simulink model "VB_RIFKF_UWB_INS25"  (R2023a)
settings: Solver=FixedStepAuto  StartTime=0.0  StopTime=500  FixedStep=0.01  RelTol=1e-3
InitFcn:
  | resilient_initNavigation1216;
  | init_param;
  | param_bias;
undefined symbols (not defined in the file or in its folder): dt, g0, gam0_rad, ISUS_flag, lp_GPS_sample_time, lp_Lidar_knoise, lp_Lidar_max, lp_Lidar_min, lp_Lidar_sample_time, lp_Lidar_seed, lp_UWB_knoise, lp_UWB_sample_time, lp_UWB_seed, lp_UWB_XY_max, lp_UWB_XY_min, magnitude, p, P0, P0_RIEKF, param, pd0, pe0, phi0_rad, pn0, psi, psi0_rad, state_dim, vd0, ve0, vn0
libraries: simulink_extras x108, simulink x89, dspstat3 x74, sharedtransform x61, matrix_library x11, sharedTrackingLibrary x8, aerolibconvert2 x5, aerolibtransform2 x5, dspfactors x3
(part 17 of 29)

== system VB_RIFKF_UWB_INS25/相对传感器模拟3/Subsystem/laser model ==
  note: 方位角测量白噪声均方根 ：0.1°
  psi & theta : Inport
  Bus Creator : BusCreator  Inputs=2
  Demux : Demux  Outputs=2
  Zero-Order Hold1 : ZeroOrderHold  SampleTime=lp_GPS_sample_time
  Zero-Order Hold2 : ZeroOrderHold  SampleTime=lp_GPS_sample_time
  bias & noise z1 : Subsystem  mask(Bias and Noise Model){noise_min=lp_Lidar_min, noise_max=lp_Lidar_max, noise_seed=lp_Lidar_seed, noise_k=lp_Lidar_knoise, sample_time=lp_Lidar_sample_time}
      mask prompts: noise_min "Minimum of the noise:"; noise_max "Maximum of the noise:"; noise_seed "Seed of the noise:"; noise_k "Noise coefficiet:"; sample_time "Sample time"
  bias & noise z3 : Subsystem  mask(Bias and Noise Model){noise_min=lp_Lidar_min, noise_max=lp_Lidar_max, noise_seed=lp_Lidar_seed, noise_k=lp_Lidar_knoise, sample_time=lp_Lidar_sample_time}
      mask prompts: noise_min "Minimum of the noise:"; noise_max "Maximum of the noise:"; noise_seed "Seed of the noise:"; noise_k "Noise coefficiet:"; sample_time "Sample time"
  psi out : Outport
  wires:
  Zero-Order Hold2/1 -> bias & noise z1/1(normal)  "theta13"
  Zero-Order Hold1/1 -> bias & noise z3/1(normal)  "theta12"
  Bus Creator/1 -> psi out/1
  bias & noise z3/1(real) -> Bus Creator/1  "psi12_k"
  bias & noise z1/1(real) -> Bus Creator/2  "psi12_k-1"
  psi & theta/1 -> Demux/1
  Demux/1 -> Zero-Order Hold1/1
  Demux/2 -> Zero-Order Hold2/1

== system VB_RIFKF_UWB_INS25/相对传感器模拟3/Subsystem2/radar model ==
  note: 相对距离测量白噪声均方根：3m
  r_xyz : Inport
  Bus Creator : BusCreator  Inputs=2
  Demux : Demux  Outputs=2
  Subsystem1 : Subsystem
  Zero-Order Hold1 : ZeroOrderHold  SampleTime=lp_GPS_sample_time
  Zero-Order Hold2 : ZeroOrderHold  SampleTime=lp_GPS_sample_time
  bias & noise x : Subsystem  mask(Bias and Noise Model){noise_min=lp_UWB_XY_min, noise_max=lp_UWB_XY_max, noise_seed=lp_UWB_seed, noise_k=lp_UWB_knoise, sample_time=lp_UWB_sample_time}
      mask prompts: noise_min "Minimum of the noise:"; noise_max "Maximum of the noise:"; noise_seed "Seed of the noise:"; noise_k "Noise coefficiet:"; sample_time "Sample time"
  bias & noise x1 : Subsystem  mask(Bias and Noise Model){noise_min=lp_UWB_XY_min, noise_max=lp_UWB_XY_max, noise_seed=lp_UWB_seed, noise_k=lp_UWB_knoise, sample_time=lp_UWB_sample_time}
      mask prompts: noise_min "Minimum of the noise:"; noise_max "Maximum of the noise:"; noise_seed "Seed of the noise:"; noise_k "Noise coefficiet:"; sample_time "Sample time"
  r_xyz out : Outport
  wires:
  Zero-Order Hold2/1 -> bias & noise x1/1(normal)  "r13"
  Zero-Order Hold1/1 -> bias & noise x/1(normal)  "r12"
  bias & noise x1/1(real) -> Subsystem1/1(u)
  bias & noise x/1(real) -> Bus Creator/1  "r12_k"
  Demux/2 -> Zero-Order Hold2/1
  Demux/1 -> Zero-Order Hold1/1
  r_xyz/1 -> Demux/1
  Bus Creator/1 -> r_xyz out/1
  Subsystem1/1(y) -> Bus Creator/2  "r12_k-1"

== system VB_RIFKF_UWB_INS25/相对传感器模拟4/Subsystem/laser model ==
  note: 方位角测量白噪声均方根 ：0.1°
  psi & theta : Inport
  Bus Creator : BusCreator  Inputs=2
  Demux : Demux  Outputs=2
  Zero-Order Hold1 : ZeroOrderHold  SampleTime=lp_GPS_sample_time
  Zero-Order Hold2 : ZeroOrderHold  SampleTime=lp_GPS_sample_time
  bias & noise z1 : Subsystem  mask(Bias and Noise Model){noise_min=lp_Lidar_min, noise_max=lp_Lidar_max, noise_seed=lp_Lidar_seed, noise_k=lp_Lidar_knoise, sample_time=lp_Lidar_sample_time}
      mask prompts: noise_min "Minimum of the noise:"; noise_max "Maximum of the noise:"; noise_seed "Seed of the noise:"; noise_k "Noise coefficiet:"; sample_time "Sample time"
  bias & noise z3 : Subsystem  mask(Bias and Noise Model){noise_min=lp_Lidar_min, noise_max=lp_Lidar_max, noise_seed=lp_Lidar_seed, noise_k=lp_Lidar_knoise, sample_time=lp_Lidar_sample_time}
      mask prompts: noise_min "Minimum of the noise:"; noise_max "Maximum of the noise:"; noise_seed "Seed of the noise:"; noise_k "Noise coefficiet:"; sample_time "Sample time"
  psi out : Outport
  wires:
  Demux/2 -> Zero-Order Hold2/1
  Demux/1 -> Zero-Order Hold1/1
  psi & theta/1 -> Demux/1
  bias & noise z1/1(real) -> Bus Creator/2  "psi12_k-1"
  bias & noise z3/1(real) -> Bus Creator/1  "psi12_k"
  Bus Creator/1 -> psi out/1
  Zero-Order Hold1/1 -> bias & noise z3/1(normal)  "theta12"
  Zero-Order Hold2/1 -> bias & noise z1/1(normal)  "theta13"

== system VB_RIFKF_UWB_INS25/相对传感器模拟4/Subsystem2/radar model ==
  note: 相对距离测量白噪声均方根：3m
  r_xyz : Inport
  Bus Creator : BusCreator  Inputs=2
  Demux : Demux  Outputs=2
  Subsystem1 : Subsystem
  Zero-Order Hold1 : ZeroOrderHold  SampleTime=lp_GPS_sample_time
  Zero-Order Hold2 : ZeroOrderHold  SampleTime=lp_GPS_sample_time
  bias & noise x : Subsystem  mask(Bias and Noise Model){noise_min=lp_UWB_XY_min, noise_max=lp_UWB_XY_max, noise_seed=lp_UWB_seed, noise_k=lp_UWB_knoise, sample_time=lp_UWB_sample_time}
      mask prompts: noise_min "Minimum of the noise:"; noise_max "Maximum of the noise:"; noise_seed "Seed of the noise:"; noise_k "Noise coefficiet:"; sample_time "Sample time"
  bias & noise x1 : Subsystem  mask(Bias and Noise Model){noise_min=lp_UWB_XY_min, noise_max=lp_UWB_XY_max, noise_seed=lp_UWB_seed, noise_k=lp_UWB_knoise, sample_time=lp_UWB_sample_time}
      mask prompts: noise_min "Minimum of the noise:"; noise_max "Maximum of the noise:"; noise_seed "Seed of the noise:"; noise_k "Noise coefficiet:"; sample_time "Sample time"
  r_xyz out : Outport
  wires:
  Subsystem1/1(y) -> Bus Creator/2  "r12_k-1"
  Bus Creator/1 -> r_xyz out/1
  r_xyz/1 -> Demux/1
  Demux/1 -> Zero-Order Hold1/1
  Demux/2 -> Zero-Order Hold2/1
  bias & noise x/1(real) -> Bus Creator/1  "r12_k"
  bias & noise x1/1(real) -> Subsystem1/1(u)
  Zero-Order Hold1/1 -> bias & noise x/1(normal)  "r12"
  Zero-Order Hold2/1 -> bias & noise x1/1(normal)  "r13"

== system VB_RIFKF_UWB_INS25/ER EKF M1/Error State Kalman Filter/Extended Kalman Filter1/Correct1 ==
  yMeas : Inport  SampleTime=SampleTime
  R : Inport  Port=2  SampleTime=SampleTime
  uMeas : Inport  Port=3  SampleTime=SampleTime
  uBlockOrdering : Inport  Port=4  SampleTime=SampleTime
  Enable : EnablePort
  Correct : MATLAB Function  TreatAsAtomicUnit=on
  Data Store ReadP : DataStoreRead  DataStoreName=P  IndexOptions=Index vector (dialog)  Indices=1  OutputSizes=1
  Data Store ReadX : DataStoreRead  DataStoreName=x  IndexOptions=Index vector (dialog)  Indices=1  OutputSizes=1
  Data Store WriteP : DataStoreWrite  DataStoreName=P  IndexOptions=Index vector (dialog)  Indices=1  OutputSizes=1
  Data Store WriteX : DataStoreWrite  DataStoreName=x  IndexOptions=Index vector (dialog)  Indices=1  OutputSizes=1
  RegisterSimulinkFcn : S-Function  FunctionName=ekfukfRegisterSimulinkFcn  Parameters=int32(3), 1, pM.HasAdditiveNoise, SampleTime, DataType, SLFcnsToRegister  SFunctionDeploymentMode=off  EnableBusSupport=off
  Scope : Scope
  Sk_m_innovation : Subsystem
  yBlockOrdering : Outport  VectorParamsAs1DForOutWhenUnconnected=off
  wires:
  Data Store ReadX/1 -> Sk_m_innovation/3(X), RegisterSimulinkFcn/1, Correct/1(x)
  Data Store ReadP/1 -> Sk_m_innovation/1(Pk/k_1), Correct/2("P ")
  Correct/2(P) -> Data Store WriteP/1
  R/1 -> Sk_m_innovation/4(R), Correct/4(R), RegisterSimulinkFcn/3
  Correct/1(xNew) -> Data Store WriteX/1
  Correct/3(blockOrdering) -> yBlockOrdering/1
  uBlockOrdering/1 -> Correct/6("blockOrdering ")
  uMeas/1 -> Correct/5(uMeas)
  yMeas/1 -> Sk_m_innovation/2(yMeas), RegisterSimulinkFcn/2, Correct/3(yMeas)
  Sk_m_innovation/1(measurement innovation) -> Scope/1

== system VB_RIFKF_UWB_INS25/ER EKF M1/Error State Kalman Filter/Extended Kalman Filter1/Output ==
  uBlockOrdering : Inport
  Data Store Read : DataStoreRead  DataStoreName=x  IndexOptions=Index vector (dialog)  Indices=1  OutputSizes=1
  Data Store Read1 : DataStoreRead  DataStoreName=P  IndexOptions=Index vector (dialog)  Indices=1  OutputSizes=1
  MATLAB Function : MATLAB Function  TreatAsAtomicUnit=on
  x : Outport  VectorParamsAs1DForOutWhenUnconnected=off
  P : Outport  Port=2  VectorParamsAs1DForOutWhenUnconnected=off
  yBlockOrdering : Outport  Port=3  VectorParamsAs1DForOutWhenUnconnected=off
  wires:
  Data Store Read/1 -> x/1
  Data Store Read1/1 -> MATLAB Function/1(S)
  uBlockOrdering/1 -> yBlockOrdering/1
  MATLAB Function/1(P) -> P/1

== system VB_RIFKF_UWB_INS25/ER EKF M1/Error State Kalman Filter/Extended Kalman Filter1/Predict ==
  Q : Inport  SampleTime=SampleTime
  uState : Inport  Port=2  SampleTime=SampleTime
  uBlockOrdering : Inport  Port=3  SampleTime=SampleTime
  Data Store Read1 : DataStoreRead  Commented=on  DataStoreName=feedback_flag_18dim  IndexOptions=Index vector (dialog)  Indices=1  OutputSizes=1
  Data Store Write : DataStoreWrite  DataStoreName=P  IndexOptions=Index vector (dialog)  Indices=1  OutputSizes=1
  Data Store Write1 : DataStoreWrite  DataStoreName=x  IndexOptions=Index vector (dialog)  Indices=1  OutputSizes=1
  Data Store WriteX : DataStoreWrite  DataStoreName=x  IndexOptions=Index vector (dialog)  Indices=1  OutputSizes=1
  Data Store ReadP : DataStoreRead  DataStoreName=P  IndexOptions=Index vector (dialog)  Indices=1  OutputSizes=1
  Data Store ReadX : DataStoreRead  DataStoreName=x  IndexOptions=Index vector (dialog)  Indices=1  OutputSizes=1
  If : If  Commented=on  IfExpression=u1 == 1  ShowElse=off
  If Action Subsystem : Subsystem  Commented=on  TreatAsAtomicUnit=on
  Predict : MATLAB Function  TreatAsAtomicUnit=on
  RegisterSimulinkFcn : S-Function  FunctionName=ekfukfRegisterSimulinkFcn  Parameters=int32(2), 0, pS.HasAdditiveNoise, SampleTime, DataType, SLFcnsToRegister  SFunctionDeploymentMode=off  EnableBusSupport=off
  Zero : Constant  Value=zeros(15,1)  OutDataTypeStr=Inherit: Inherit via back propagation
  wires:
  Data Store ReadP/1 -> Predict/2("P ")
  Predict/2(P) -> Data Store Write/1
  Q/1 -> Predict/3(Q), RegisterSimulinkFcn/2
  Predict/1(xNew) -> Data Store WriteX/1
  Data Store ReadX/1 -> Predict/1(x), RegisterSimulinkFcn/1
  uBlockOrdering/1 -> Predict/5(unused)
  uState/1 -> Predict/4(uState)
  Data Store Read1/1 -> If/1
  If/1 -> If Action Subsystem/Action
  Zero/1 -> Data Store Write1/1

== system VB_RIFKF_UWB_INS25/ER EKF M1/Error State Kalman Filter/Simulink Function - State Transition/Cal Phi ==
  <DCM_b_n> : Inport
  wxyz : Inport  Port=2
  axyz : Inport  Port=3
  Constant : Constant  Value=dt
  MATLAB Function1 : MATLAB Function  TreatAsAtomicUnit=on
  Transpose : Math  Operator=transpose
  Phi : Outport
  wires:
  <DCM_b_n>/1 -> Transpose/1
  MATLAB Function1/1(Phi) -> Phi/1
  wxyz/1 -> MATLAB Function1/3(wxyz)
  axyz/1 -> MATLAB Function1/1(axyz)
  Constant/1 -> MATLAB Function1/4(dt)
  Transpose/1 -> MATLAB Function1/2(Cnb)

== system VB_RIFKF_UWB_INS25/ER EKF M1/Error State Kalman Filter/Simulink Function - State Transition Jacobian/Cal Phi1 ==
  <DCM_b_n> : Inport
  wxyz : Inport  Port=2
  axyz : Inport  Port=3
  Constant : Constant  Value=dt
  MATLAB Function1 : MATLAB Function  TreatAsAtomicUnit=on
  Transpose : Math  Operator=transpose
  Phi : Outport
  wires:
  <DCM_b_n>/1 -> Transpose/1
  MATLAB Function1/1(Phi) -> Phi/1
  wxyz/1 -> MATLAB Function1/3(wxyz)
  axyz/1 -> MATLAB Function1/1(axyz)
  Constant/1 -> MATLAB Function1/4(dt)
  Transpose/1 -> MATLAB Function1/2(Cnb)

== system VB_RIFKF_UWB_INS25/ER EKF M1/INS propogation/Init_PVQ/Horizontal_attitude ==
  note: gamma
  note: fai
  accl_mean_B_m/s_LPF : Inport  PortDimensions=3
  Magn_mean_B_guess_LPF : Inport  Port=2
  Enable : EnablePort
  Add : Sum  Inputs=+-
  Add1 : Sum
  Add2 : Sum
  Add3 : Sum
  Asin : Trigonometry  Operator=asin
  Atan2 : Trigonometry  Operator=atan2
  Data Type Conversion : DataTypeConversion  SaturateOnIntegerOverflow=off  RndMeth=Floor
  Deal with zero : Subsystem
  Degrees to Radians : simulink_extras/Transformations/Degrees to Radians
  Degrees to Radians1 : simulink_extras/Transformations/Degrees to Radians
  Demux : Demux  Outputs=3
  Divide : Product  Inputs=*/  OutDataTypeStr=single
  Gain1 : Gain  Gain=-1
  Gain2 : Gain  Gain=-1
  Hem2JPL : MATLAB Function  TreatAsAtomicUnit=on
  Hem2JPL1 : MATLAB Function  TreatAsAtomicUnit=on
  Magnetic declination : Constant  Value=param.fusion.magDeclDeg  OutDataTypeStr=single
  Magnetic declination1 : Constant  Value=param.control.MagnheadingCorrection  OutDataTypeStr=uint8
  Math Function : Math  Operator=magnitude^2  SignedPower=on
  Mux : Mux  Inputs=3
  Mux1 : Mux  Inputs=3
  Mux3 : Mux  Inputs=3
  Product : Product  Multiplication=Matrix(*)
  Quaternions to Direction Cosine Matrix : sharedtransform/Quaternions to  Direction Cosine Matrix  aMode=aMode
  Rotation Angles to Quaternions : sharedtransform/Rotation Angles to Quaternions  rotationOrder=ZYX  aMode=aMode
  Rotation Angles to Quaternions1 : sharedtransform/Rotation Angles to Quaternions  rotationOrder=ZYX  aMode=aMode
  Scope : Scope
  Scope1 : Scope
  Selector : Selector  InputPortWidth=3  IndexOptions=Index vector (dialog)  Indices=[2]  OutputSizes=1
  Selector1 : Selector  InputPortWidth=3  IndexOptions=Index vector (dialog)  Indices=[1]  OutputSizes=1
  Sqrt : Sqrt
  Sum of Elements : Sum  Inputs=+
  Switch : Switch  Threshold=0.5  SaturateOnIntegerOverflow=off  InputSameDT=off
  Terminator : Terminator
  Transpose : Math  Operator=transpose  SignedPower=on
  Trigonometric Function1 : Trigonometry  Operator=atan2
  psi_zero : Constant  Value=psi  OutDataTypeStr=single
  psi_zero1 : Constant  Value=psi0_rad  OutDataTypeStr=single
  psi_zero2 : Constant  Value=phi0_rad  OutDataTypeStr=single
  psi_zero3 : Constant  Value=gam0_rad  OutDataTypeStr=single
  quat_0 : Outport  PortDimensions=4
  wires:
  Data Type Conversion/1 -> Scope/1
  Rotation Angles to Quaternions1/1 -> Hem2JPL1/1(q)
  Switch/1 -> quat_0/1, Scope1/1
  Magnetic declination1/1 -> Switch/2, Data Type Conversion/1
  Degrees to Radians/1 -> Terminator/1
  Add1/1 -> Mux1/1
  Gain1/1 -> Mux/3, Trigonometric Function1/2
  Transpose/1 -> Product/1
  Mux3/1 -> Rotation Angles to Quaternions1/1
  Add/1 -> Mux3/1  "psi_calbymag"
  Magnetic declination/1 -> Degrees to Radians/1
  Atan2/1 -> Add/2
  Selector/1 -> Atan2/1  "magE"
  Selector1/1 -> Atan2/2  "magN"
  Product/1 -> Selector1/1, Selector/1  "magNED"
  Magn_mean_B_guess_LPF/1 -> Product/2
  Quaternions to Direction Cosine Matrix/1 -> Transpose/1
  Rotation Angles to Quaternions/1 -> Hem2JPL/1(q)  "q0_no_yaw"
  Add3/1 -> Mux3/3, Mux1/3
  Add2/1 -> Mux1/2, Mux3/2
  psi_zero/1 -> Degrees to Radians1/1
  Mux1/1 -> Rotation Angles to Quaternions/1
  Math Function/1 -> Sum of Elements/1
  Mux/1 -> Math Function/1
  Divide/1 -> Asin/1
  Sum of Elements/1 -> Sqrt/1
  Demux/3 -> Gain1/1
  Demux/2 -> Trigonometric Function1/1, Mux/1
  Demux/1 -> Mux/2, Divide/1
  Trigonometric Function1/1 -> Gain2/1
  Deal with zero/1(Out1) -> Divide/2
  Sqrt/1 -> Deal with zero/1(In1)
  accl_mean_B_m/s_LPF/1 -> Demux/1
  Hem2JPL/1(y) -> Switch/1, Quaternions to Direction Cosine Matrix/1, Switch/3
  Degrees to Radians1/1 -> Add1/2
  psi_zero1/1 -> Add1/1
  Asin/1 -> Add2/2
  psi_zero2/1 -> Add2/1
  Gain2/1 -> Add3/2
  psi_zero3/1 -> Add3/1

== system VB_RIFKF_UWB_INS25/ER EKF M1/INS propogation/Init_PVQ/Horizontal_attitude2 ==
  note: gamma
  note: fai
  accl_mean_B_m/s_LPF : Inport  PortDimensions=3
  Magn_mean_B_guess_LPF : Inport  Port=2
  Enable : EnablePort
  Add : Sum  Inputs=+-
  Add1 : Sum
  Add2 : Sum
  Asin : Trigonometry  Operator=asin
  Atan2 : Trigonometry  Operator=atan2
  Data Type Conversion : DataTypeConversion  SaturateOnIntegerOverflow=off  RndMeth=Floor
  Deal with zero : Subsystem
  Degrees to Radians : simulink_extras/Transformations/Degrees to Radians
  Degrees to Radians1 : simulink_extras/Transformations/Degrees to Radians
  Demux : Demux  Outputs=3
  Display : Display
  Divide : Product  Inputs=*/  OutDataTypeStr=single
  Gain1 : Gain  Gain=-1
  Gain2 : Gain  Gain=-1
  Hem2JPL1 : MATLAB Function  TreatAsAtomicUnit=on
  Hem2JPL2 : MATLAB Function  TreatAsAtomicUnit=on
  Magnetic declination : Constant  Value=param.fusion.magDeclDeg  OutDataTypeStr=single
  Magnetic declination1 : Constant  Value=param.control.MagnheadingCorrection  OutDataTypeStr=uint8
  Math Function : Math  Operator=magnitude^2  SignedPower=on
  Mux : Mux  Inputs=3
  Mux1 : Mux  Inputs=3
  Mux3 : Mux  Inputs=3
  Product : Product  Multiplication=Matrix(*)
  Quaternions to Direction Cosine Matrix : sharedtransform/Quaternions to  Direction Cosine Matrix  aMode=aMode
  Radians to Degrees : simulink_extras/Transformations/Radians to Degrees
  Rotation Angles to Quaternions : sharedtransform/Rotation Angles to Quaternions  rotationOrder=ZYX  aMode=aMode
  Rotation Angles to Quaternions1 : sharedtransform/Rotation Angles to Quaternions  rotationOrder=ZYX  aMode=aMode
  Scope : Scope
  Scope1 : Scope
  Selector : Selector  InputPortWidth=3  IndexOptions=Index vector (dialog)  Indices=[2]  OutputSizes=1
  Selector1 : Selector  InputPortWidth=3  IndexOptions=Index vector (dialog)  Indices=[1]  OutputSizes=1
  Sqrt : Sqrt
  Sum of Elements : Sum  Inputs=+
  Switch : Switch  Threshold=0.5  SaturateOnIntegerOverflow=off  InputSameDT=off
  Terminator : Terminator
  Transpose : Math  Operator=transpose  SignedPower=on
  Trigonometric Function1 : Trigonometry  Operator=atan2
  phi0_rad : Constant  Value=phi0_rad  OutDataTypeStr=single
  phi0_rad1 : Constant  Value=gam0_rad  OutDataTypeStr=single
  psi_zero : Constant  Value=psi  OutDataTypeStr=single
  psi_zero1 : Constant  Commented=on  Value=psi  OutDataTypeStr=single
  quat_0 : Outport  PortDimensions=4
  wires:
  Rotation Angles to Quaternions1/1 -> Hem2JPL1/1(q)
  Hem2JPL2/1(y) -> Quaternions to Direction Cosine Matrix/1, Switch/3
  Hem2JPL1/1(y) -> Switch/1
  Gain2/1 -> Add2/2
  phi0_rad1/1 -> Add2/1
  phi0_rad/1 -> Add1/1
  Asin/1 -> Add1/2
  Radians to Degrees/1 -> Display/1
  Data Type Conversion/1 -> Scope/1
  Switch/1 -> quat_0/1, Scope1/1
  Magnetic declination1/1 -> Switch/2, Data Type Conversion/1
  Degrees to Radians/1 -> Terminator/1
  Degrees to Radians1/1 -> Mux1/1, Radians to Degrees/1
  Gain1/1 -> Mux/3, Trigonometric Function1/2
  Transpose/1 -> Product/1
  Mux3/1 -> Rotation Angles to Quaternions1/1
  Add/1 -> Mux3/1  "psi_calbymag"
  Magnetic declination/1 -> Degrees to Radians/1
  Atan2/1 -> Add/2
  Selector/1 -> Atan2/1  "magE"
  Selector1/1 -> Atan2/2  "magN"
  Product/1 -> Selector1/1, Selector/1  "magNED"
  Magn_mean_B_guess_LPF/1 -> Product/2
  Quaternions to Direction Cosine Matrix/1 -> Transpose/1
  Rotation Angles to Quaternions/1 -> Hem2JPL2/1(q)  "q0_no_yaw"
  Add2/1 -> Mux1/3, Mux3/3
  Add1/1 -> Mux1/2, Mux3/2
  psi_zero/1 -> Degrees to Radians1/1
  Mux1/1 -> Rotation Angles to Quaternions/1
  Math Function/1 -> Sum of Elements/1
  Mux/1 -> Math Function/1
  Divide/1 -> Asin/1
  Sum of Elements/1 -> Sqrt/1
  Demux/3 -> Gain1/1
  Demux/2 -> Trigonometric Function1/1, Mux/1
  Demux/1 -> Mux/2, Divide/1
  Trigonometric Function1/1 -> Gain2/1
  Deal with zero/1(Out1) -> Divide/2
  Sqrt/1 -> Deal with zero/1(In1)
  accl_mean_B_m/s_LPF/1 -> Demux/1

== system VB_RIFKF_UWB_INS25/ER EKF M1/INS propogation/Init_PVQ/Subsystem ==
  data : Inport
  Buffer : Buffer  N=50  V=49  OutputFrames=off
  Buffer1 : Buffer  N=50  V=49  OutputFrames=off
  Buffer2 : Buffer  N=50  V=49  ic=-g0  OutputFrames=off
  Demux : Demux  Outputs=3
  Mean4 : dspstat3/Mean  run=off  reset_popup=None  directionMode=Entire input  dimension=3  roiEnable=off  roiType=Rectangles  roiPortion=Entire ROI  roiOutput=Individual statistics for each ROI  roiFlag=off  roundingMode=Floor  overflowMode=off  outputDataTypeStr=Inherit: Same as accumulator  outputMin=[]  outputMax=[]  outputLastDataTypeStr=Inherit: Same as accumulator
  Mean5 : dspstat3/Mean  run=off  reset_popup=None  directionMode=Entire input  dimension=3  roiEnable=off  roiType=Rectangles  roiPortion=Entire ROI  roiOutput=Individual statistics for each ROI  roiFlag=off  roundingMode=Floor  overflowMode=off  outputDataTypeStr=Inherit: Same as accumulator  outputMin=[]  outputMax=[]  outputLastDataTypeStr=Inherit: Same as accumulator
  Mean6 : dspstat3/Mean  run=off  reset_popup=None  directionMode=Entire input  dimension=3  roiEnable=off  roiType=Rectangles  roiPortion=Entire ROI  roiOutput=Individual statistics for each ROI  roiFlag=off  roundingMode=Floor  overflowMode=off  outputDataTypeStr=Inherit: Same as accumulator  outputMin=[]  outputMax=[]  outputLastDataTypeStr=Inherit: Same as accumulator
  Scope : Scope  NumInputPorts=2
  Vector Concatenate : Concatenate  NumInputs=3
  mean_data : Outport
  wires:
  data/1 -> Demux/1, Scope/1
  Vector Concatenate/1 -> mean_data/1, Scope/2
  Mean4/1 -> Vector Concatenate/1
  Demux/3 -> Buffer2/1
  Buffer1/1 -> Mean5/1  "fby_buff"
  Demux/1 -> Buffer/1
  Buffer2/1 -> Mean6/1  "fbz_buff"
  Mean5/1 -> Vector Concatenate/2
  Buffer/1 -> Mean4/1  "fbx_buff"
  Demux/2 -> Buffer1/1
  Mean6/1 -> Vector Concatenate/3

== system VB_RIFKF_UWB_INS25/ER EKF M1/INS propogation/Init_PVQ/Subsystem1 ==
  data : Inport
  Buffer : Buffer  N=50  V=49  OutputFrames=off
  Buffer1 : Buffer  N=50  V=49  OutputFrames=off
  Buffer2 : Buffer  N=50  V=49  OutputFrames=off
  Demux : Demux  Outputs=3
  Mean4 : dspstat3/Mean  run=off  reset_popup=None  directionMode=Entire input  dimension=3  roiEnable=off  roiType=Rectangles  roiPortion=Entire ROI  roiOutput=Individual statistics for each ROI  roiFlag=off  roundingMode=Floor  overflowMode=off  outputDataTypeStr=Inherit: Same as accumulator  outputMin=[]  outputMax=[]  outputLastDataTypeStr=Inherit: Same as accumulator
  Mean5 : dspstat3/Mean  run=off  reset_popup=None  directionMode=Entire input  dimension=3  roiEnable=off  roiType=Rectangles  roiPortion=Entire ROI  roiOutput=Individual statistics for each ROI  roiFlag=off  roundingMode=Floor  overflowMode=off  outputDataTypeStr=Inherit: Same as accumulator  outputMin=[]  outputMax=[]  outputLastDataTypeStr=Inherit: Same as accumulator
  Mean6 : dspstat3/Mean  run=off  reset_popup=None  directionMode=Entire input  dimension=3  roiEnable=off  roiType=Rectangles  roiPortion=Entire ROI  roiOutput=Individual statistics for each ROI  roiFlag=off  roundingMode=Floor  overflowMode=off  outputDataTypeStr=Inherit: Same as accumulator  outputMin=[]  outputMax=[]  outputLastDataTypeStr=Inherit: Same as accumulator
  Vector Concatenate : Concatenate  NumInputs=3
  mean_data : Outport
  wires:
  Mean6/1 -> Vector Concatenate/3
  Demux/2 -> Buffer1/1
  Buffer/1 -> Mean4/1  "fbx_buff"
  Mean5/1 -> Vector Concatenate/2
  Buffer2/1 -> Mean6/1  "fbz_buff"
  Demux/1 -> Buffer/1
  Buffer1/1 -> Mean5/1  "fby_buff"
  Demux/3 -> Buffer2/1
  Mean4/1 -> Vector Concatenate/1
  Vector Concatenate/1 -> mean_data/1
  data/1 -> Demux/1

== system VB_RIFKF_UWB_INS25/ER EKF M1/INS propogation/accl bias compensation/error compensation1 ==
  dda : Inport
  Add3 : Sum
  Memory1 : Memory
  da : Outport
  wires:
  Memory1/1 -> Add3/2
  Add3/1 -> Memory1/1, da/1
  dda/1 -> Add3/1

== system VB_RIFKF_UWB_INS25/ER EKF M1/INS propogation/gyro bias compensation/error compensation ==
  ddg : Inport
  Enable : Inport  Port=2
  Add3 : Sum
  Data Store Read5 : DataStoreRead  DataStoreName=GPS_enable  IndexOptions=Index vector (dialog)  Indices=1  OutputSizes=1
  If Action Subsystem1 : Subsystem  TreatAsAtomicUnit=on
  If1 : If  IfExpression=u1 == 1  ShowElse=off
  Memory1 : Memory
  Scope : Scope
  dg : Outport
  wires:
  ddg/1 -> Add3/1
  Add3/1 -> Memory1/1, dg/1
  Memory1/1 -> Add3/2
  If1/1 -> If Action Subsystem1/Action
  Enable/1 -> If1/1, Scope/1

== system VB_RIFKF_UWB_INS25/ER EKF M1/INS propogation/vel_pos_update/Kinematic Equation ==
  Cbn : Inport
  Ab : Inport  Port=2
  Add : Sum  Inputs=+-
  Constant : Constant  Value=[0 0 -g0]  OutDataTypeStr=single
  Product : Product  Multiplication=Matrix(*)  RndMeth=Zero
  Scope : Scope
  Scope1 : Scope  NumInputPorts=2
  An : Outport
  wires:
  Constant/1 -> Add/2
  Product/1 -> Add/1, Scope/1
  Ab/1 -> Scope1/1, Product/2
  Add/1 -> Scope1/2, An/1
  Cbn/1 -> Product/1

== system VB_RIFKF_UWB_INS25/ER EKF M1/INS propogation/vel_pos_update/pos update ==
  vel_k : Inport
  dp : Inport  Port=2
  QGC_init : Inport  Port=3
  p0 : Inport  Port=4
  Add1 : Sum  Inputs=++-
  Data Store Read2 : DataStoreRead  DataStoreName=GPS_enable  IndexOptions=Index vector (dialog)  Indices=1  OutputSizes=1
  Delay1 : Delay  DelayLength=1  InitialConditionSource=Input port  ExternalReset=Rising
      settings: InputPortMap=u0,r5,p4
  Gain1 : Gain  Gain=dt
  Memory : Memory
  Product : Product
  Reshape1 : Reshape  OutputDimensionality=Column vector (2-D)
  p_k : Outport
  wires:
  Memory/1 -> Product/2
  Data Store Read2/1 -> Memory/1
  dp/1 -> Product/1, Add1/3
  vel_k/1 -> Gain1/1
  Gain1/1 -> Add1/1
  Delay1/1 -> Add1/2
  Reshape1/1 -> Delay1/3
  Add1/1 -> p_k/1, Delay1/1
  QGC_init/1 -> Delay1/2
  p0/1 -> Reshape1/1

== system VB_RIFKF_UWB_INS25/ER EKF M1/INS propogation/vel_pos_update/vel update ==
  QGC_init : Inport
  An : Inport  Port=2
  KFState_dv : Inport  Port=3
  v0 : Inport  Port=4
  Add : Sum  Inputs=++-
  Data Store Read2 : DataStoreRead  DataStoreName=GPS_enable  IndexOptions=Index vector (dialog)  Indices=1  OutputSizes=1
  Delay : Delay  DelayLength=1  InitialConditionSource=Input port  ExternalReset=Rising
      settings: InputPortMap=u0,r5,p4
  Gain : Gain  Gain=dt
  Memory : Memory
  Product : Product
  Reshape : Reshape  OutputDimensionality=Column vector (2-D)
  Scope : Scope  NumInputPorts=3
  vel_k : Outport
  wires:
  Memory/1 -> Product/2, Scope/3
  KFState_dv/1 -> Product/1, Add/3, Scope/2, Scope/1
  Data Store Read2/1 -> Memory/1
  Delay/1 -> Add/2
  Gain/1 -> Add/1
  Add/1 -> vel_k/1, Delay/1
  v0/1 -> Reshape/1
  An/1 -> Gain/1
  Reshape/1 -> Delay/3
  QGC_init/1 -> Delay/2

== system VB_RIFKF_UWB_INS25/ISUS_RIEKF M1/Error State Kalman Filter M1/Extended Kalman Filter M1/Correct M1 ==
  yMeas : Inport  SampleTime=SampleTime
  R : Inport  Port=2  SampleTime=SampleTime
  uMeas : Inport  Port=3  SampleTime=SampleTime
  uBlockOrdering : Inport  Port=4  SampleTime=SampleTime
  Enable : EnablePort
  Correct : MATLAB Function  TreatAsAtomicUnit=on
  Data Store Read : DataStoreRead  DataStoreName=x  IndexOptions=Index vector (dialog)  Indices=1  OutputSizes=1
  Data Store Read1 : DataStoreRead  DataStoreName=P  IndexOptions=Index vector (dialog)  Indices=1  OutputSizes=1
  Data Store Write2 : DataStoreWrite  Commented=on  DataStoreName=x  IndexOptions=Index vector (dialog)  Indices=1  OutputSizes=1
  Data Store Write3 : DataStoreWrite  Commented=on  DataStoreName=P  IndexOptions=Index vector (dialog)  Indices=1  OutputSizes=1
  Data Store WriteP : DataStoreWrite  DataStoreName=P  IndexOptions=Index vector (dialog)  Indices=1  OutputSizes=1
  Data Store WriteX : DataStoreWrite  DataStoreName=x  IndexOptions=Index vector (dialog)  Indices=1  OutputSizes=1
  RegisterSimulinkFcn : S-Function  FunctionName=ekfukfRegisterSimulinkFcn  Parameters=int32(3), 1, pM.HasAdditiveNoise, SampleTime, DataType, SLFcnsToRegister  SFunctionDeploymentMode=off  EnableBusSupport=off
  Scope : Scope
  yBlockOrdering : Outport  VectorParamsAs1DForOutWhenUnconnected=off
  wires:
  Correct/2(P) -> Data Store WriteP/1
  Data Store Read1/1 -> Correct/2("P ")
  Data Store Read/1 -> RegisterSimulinkFcn/1, Correct/1(x)
  yMeas/1 -> Correct/3(yMeas), RegisterSimulinkFcn/2, Scope/1
  R/1 -> Correct/4(R), RegisterSimulinkFcn/3
  Correct/1(xNew) -> Data Store WriteX/1
  Correct/3(blockOrdering) -> yBlockOrdering/1
  uBlockOrdering/1 -> Correct/6("blockOrdering ")
  uMeas/1 -> Correct/5(uMeas)

== system VB_RIFKF_UWB_INS25/ISUS_RIEKF M1/Error State Kalman Filter M1/Extended Kalman Filter M1/Output ==
  uBlockOrdering : Inport
  Data Store Read : DataStoreRead  DataStoreName=x  IndexOptions=Index vector (dialog)  Indices=1  OutputSizes=1
  Data Store Read1 : DataStoreRead  DataStoreName=P  IndexOptions=Index vector (dialog)  Indices=1  OutputSizes=1
  MATLAB Function : MATLAB Function  TreatAsAtomicUnit=on
  x : Outport  VectorParamsAs1DForOutWhenUnconnected=off
  P : Outport  Port=2  VectorParamsAs1DForOutWhenUnconnected=off
  yBlockOrdering : Outport  Port=3  VectorParamsAs1DForOutWhenUnconnected=off
  wires:
  MATLAB Function/1(P) -> P/1
  Data Store Read1/1 -> MATLAB Function/1(S)
  Data Store Read/1 -> x/1
  uBlockOrdering/1 -> yBlockOrdering/1

== system VB_RIFKF_UWB_INS25/ISUS_RIEKF M1/Error State Kalman Filter M1/Extended Kalman Filter M1/Predict ==
  Q : Inport  SampleTime=SampleTime
  uState : Inport  Port=2  SampleTime=SampleTime
  uBlockOrdering : Inport  Port=3  SampleTime=SampleTime
  Data Store Read1 : DataStoreRead  Commented=on  DataStoreName=feedback_flag_18dim  IndexOptions=Index vector (dialog)  Indices=1  OutputSizes=1
  Data Store Write : DataStoreWrite  DataStoreName=P  IndexOptions=Index vector (dialog)  Indices=1  OutputSizes=1
  Data Store Write1 : DataStoreWrite  DataStoreName=x  IndexOptions=Index vector (dialog)  Indices=1  OutputSizes=1
  Data Store WriteX : DataStoreWrite  DataStoreName=x  IndexOptions=Index vector (dialog)  Indices=1  OutputSizes=1
  Data Store ReadP : DataStoreRead  DataStoreName=P  IndexOptions=Index vector (dialog)  Indices=1  OutputSizes=1
  Data Store ReadX : DataStoreRead  DataStoreName=x  IndexOptions=Index vector (dialog)  Indices=1  OutputSizes=1
  If : If  Commented=on  IfExpression=u1 == 1  ShowElse=off
  If Action Subsystem : Subsystem  Commented=on  TreatAsAtomicUnit=on
  Predict : MATLAB Function  TreatAsAtomicUnit=on
  RegisterSimulinkFcn : S-Function  FunctionName=ekfukfRegisterSimulinkFcn  Parameters=int32(2), 0, pS.HasAdditiveNoise, SampleTime, DataType, SLFcnsToRegister  SFunctionDeploymentMode=off  EnableBusSupport=off
  Zero : Constant  Value=zeros(state_dim,1)  OutDataTypeStr=Inherit: Inherit via back propagation
  wires:
  Data Store ReadP/1 -> Predict/2("P ")
  Predict/2(P) -> Data Store Write/1
  Q/1 -> Predict/3(Q), RegisterSimulinkFcn/2
  Predict/1(xNew) -> Data Store WriteX/1
  Data Store ReadX/1 -> Predict/1(x), RegisterSimulinkFcn/1
  uBlockOrdering/1 -> Predict/5(unused)
  uState/1 -> Predict/4(uState)
  Data Store Read1/1 -> If/1
  If/1 -> If Action Subsystem/Action
  Zero/1 -> Data Store Write1/1

== system VB_RIFKF_UWB_INS25/ISUS_RIEKF M1/Error State Kalman Filter M1/Simulink Function - State Transition/Cal Phi ==
  Rbn : Inport
  vn : Inport  Port=2
  pn : Inport  Port=3
  Constant : Constant  Value=dt
  MATLAB Function1 : MATLAB Function  TreatAsAtomicUnit=on
  Reshape : Reshape  OutputDimensionality=Column vector (2-D)
  Reshape1 : Reshape  OutputDimensionality=Column vector (2-D)
  Phi : Outport
  wires:
  Reshape1/1 -> MATLAB Function1/2(pn)
  Reshape/1 -> MATLAB Function1/1(vn)
  pn/1 -> Reshape1/1
  vn/1 -> Reshape/1
  Rbn/1 -> MATLAB Function1/3(Rbn)
  MATLAB Function1/1(Phi) -> Phi/1
  Constant/1 -> MATLAB Function1/4(dt)

== system VB_RIFKF_UWB_INS25/ISUS_RIEKF M1/Error State Kalman Filter M1/Simulink Function - State Transition1/Cal Phi ==
  Rbn : Inport
  vn : Inport  Port=2
  pn : Inport  Port=3
  Constant : Constant  Value=dt  OutDataTypeStr=single
  MATLAB Function1 : MATLAB Function  TreatAsAtomicUnit=on
  Reshape : Reshape  OutputDimensionality=Column vector (2-D)
  Reshape1 : Reshape  OutputDimensionality=Column vector (2-D)
  Phi : Outport
  wires:
  Constant/1 -> MATLAB Function1/4(dt)
  MATLAB Function1/1(Phi) -> Phi/1
  Rbn/1 -> MATLAB Function1/3(Rbn)
  vn/1 -> Reshape/1
  pn/1 -> Reshape1/1
  Reshape/1 -> MATLAB Function1/1(vn)
  Reshape1/1 -> MATLAB Function1/2(pn)

== system VB_RIFKF_UWB_INS25/ISUS_RIEKF M1/Error State Kalman Filter M1/bak/Simulink Function - GPS Measurements1 ==
  DCM_b_n : Inport
  DynamicMeasurementFcn_Dyn : TriggerPort  TriggerType=function-call  IsSimulinkFunction=on  FunctionName=DynamicMeasurementFcn_Dyn  VariantControl=Variant
  Add : Sum  Commented=on
  Add1 : Sum
  Constant : Constant  Commented=on  Value=dt  OutDataTypeStr=single
  Constant6 : Constant  Value=[zeros(3,3),eye(3),zeros(3,12);zeros(3,15),eye(3)]  OutDataTypeStr=single
  Data Type Conversion6 : DataTypeConversion  Commented=on  OutDataTypeStr=single  SaturateOnIntegerOverflow=off  RndMeth=Floor
  From7 : From  Commented=on  GotoTag=DCM_b_n
  Goto : Goto  Commented=on  GotoTag=DCM_b_n
  MATLAB Function1 : MATLAB Function  Commented=on  TreatAsAtomicUnit=on
  Product : Product  Commented=on  Multiplication=Matrix(*)
  Product1 : Product  Multiplication=Matrix(*)
  x : ArgIn  DisableCoverage=on  OutDataTypeStr=single  PortDimensions=18  ArgumentName=x
  v : ArgIn  DisableCoverage=on  Port=2  OutDataTypeStr=single  PortDimensions=6  ArgumentName=v
  y : ArgOut  DisableCoverage=on  OutDataTypeStr=single  PortDimensions=6  ArgumentName=y
  wires:
  x/1 -> Product1/2
  Constant6/1 -> Product1/1
  Product1/1 -> Add1/1
  v/1 -> Add1/2
  Add1/1 -> y/1
  Data Type Conversion6/1 -> Product/1
  DCM_b_n/1 -> Goto/1
  Constant/1 -> MATLAB Function1/2(dt)
  From7/1 -> MATLAB Function1/1(Cbn)
  MATLAB Function1/1(H) -> Data Type Conversion6/1
  Product/1 -> Add/1

== system VB_RIFKF_UWB_INS25/ISUS_RIEKF M1/Error State Kalman Filter M1/bak/Simulink Function - GPS Measurements2 ==
  ZUPTMeasurementFcn2 : TriggerPort  TriggerType=function-call  IsSimulinkFunction=on  FunctionName=ZUPTMeasurementFcn2  VariantControl=Variant
  Add : Sum
  Constant6 : Constant  Value=[zeros(3,3),eye(3),zeros(3,12)]  OutDataTypeStr=single
  Product : Product  Multiplication=Matrix(*)
  x : ArgIn  DisableCoverage=on  OutDataTypeStr=single  PortDimensions=18  ArgumentName=x
  v : ArgIn  DisableCoverage=on  Port=2  OutDataTypeStr=single  PortDimensions=3  ArgumentName=v
  y : ArgOut  DisableCoverage=on  OutDataTypeStr=single  PortDimensions=3  ArgumentName=y
  wires:
  v/1 -> Add/2
  Constant6/1 -> Product/1
  x/1 -> Product/2
  Product/1 -> Add/1
  Add/1 -> y/1

== system VB_RIFKF_UWB_INS25/ISUS_RIEKF M1/Error State Kalman Filter M1/bak/Simulink Function - State Transition Jacobian ==
  DCM_b_n : Inport
  vn : Inport  Port=2
  pn : Inport  Port=3
  stateTransitionJacobianFcn_Dyn : TriggerPort  TriggerType=function-call  IsSimulinkFunction=on  FunctionName=stateTransitionJacobianFcn_Dyn  VariantControl=Variant
  Cal Phi1 : Subsystem
  Constant : Constant  Value=0.01  OutDataTypeStr=single
  Data Type Conversion1 : DataTypeConversion  OutDataTypeStr=single  SaturateOnIntegerOverflow=off  RndMeth=Floor
  Data Type Conversion6 : DataTypeConversion  OutDataTypeStr=single  SaturateOnIntegerOverflow=off  RndMeth=Floor
  MATLAB Function1 : MATLAB Function  TreatAsAtomicUnit=on
  Product : Product  Multiplication=Matrix(*)
  Terminator : Terminator
  Terminator1 : Terminator
  Transpose : Math  Operator=transpose
  x : ArgIn  DisableCoverage=on  OutDataTypeStr=single  PortDimensions=15  ArgumentName=x
  w : ArgIn  Port=2  OutDataTypeStr=single  PortDimensions=12  ArgumentName=w
  A : ArgOut  DisableCoverage=on  OutDataTypeStr=single  PortDimensions=[15 15]  ArgumentName=A
  G : ArgOut  Port=2  OutDataTypeStr=single  PortDimensions=[15 12]  ArgumentName=G
  wires:
  Data Type Conversion1/1 -> Product/2
  Product/1 -> G/1
  [pn] -> MATLAB Function1/3(pn)
  [vn] -> MATLAB Function1/2(vn)
  Data Type Conversion6/1 -> A/1, Product/1
  Constant/1 -> MATLAB Function1/4(dt)
  Transpose/1 -> MATLAB Function1/1(Rbn)
  [DCM_b_n] -> Transpose/1
  [DCM_b_n] -> Cal Phi1/1(Rbn)
  [pn] -> Cal Phi1/3(pn)
  [vn] -> Cal Phi1/2(vn)
  vn/1 -> [vn]
  pn/1 -> [pn]
  DCM_b_n/1 -> [DCM_b_n]
  Cal Phi1/1(Phi) -> Data Type Conversion6/1
  w/1 -> Terminator1/1
  x/1 -> Terminator/1
  MATLAB Function1/1(G) -> Data Type Conversion1/1

== system VB_RIFKF_UWB_INS25/ISUS_RIEKF M1/INS propogation/Init_PVQ/Horizontal_attitude ==
  note: gamma
  note: fai
  accl_mean_B_m/s_LPF : Inport  PortDimensions=3
  Magn_mean_B_guess_LPF : Inport  Port=2
  Enable : EnablePort
  Add : Sum  Commented=on  Inputs=+-
  Add1 : Sum
  Add2 : Sum
  Asin : Trigonometry  Operator=asin
  Atan2 : Trigonometry  Commented=on  Operator=atan2
  Data Type Conversion : DataTypeConversion  SaturateOnIntegerOverflow=off  RndMeth=Floor
  Deal with zero : Subsystem
  Degrees to Radians : simulink_extras/Transformations/Degrees to Radians  Commented=on
  Degrees to Radians1 : simulink_extras/Transformations/Degrees to Radians
  Demux : Demux  Outputs=3
  Display : Display
  Divide : Product  Inputs=*/  OutDataTypeStr=single
  Gain1 : Gain  Gain=-1
  Gain2 : Gain  Gain=-1
  Magnetic declination : Constant  Commented=on  Value=param.fusion.magDeclDeg  OutDataTypeStr=single
  Magnetic declination1 : Constant  Value=param.control.MagnheadingCorrection  OutDataTypeStr=uint8
  Math Function : Math  Operator=magnitude^2  SignedPower=on
  Mux : Mux  Inputs=3
  Mux1 : Mux  Inputs=3
  Mux3 : Mux  Commented=on  Inputs=3
  Product : Product  Commented=on  Multiplication=Matrix(*)
  Quaternions to Direction Cosine Matrix : sharedtransform/Quaternions to  Direction Cosine Matrix  Commented=on  aMode=aMode
  Radians to Degrees : simulink_extras/Transformations/Radians to Degrees  Commented=on
  Rotation Angles to Quaternions : sharedtransform/Rotation Angles to Quaternions  rotationOrder=ZYX  aMode=aMode
  Rotation Angles to Quaternions1 : sharedtransform/Rotation Angles to Quaternions  Commented=on  rotationOrder=ZYX  aMode=aMode
  Scope : Scope
  Scope1 : Scope
  Selector : Selector  Commented=on  InputPortWidth=3  IndexOptions=Index vector (dialog)  Indices=[2]  OutputSizes=1
  Selector1 : Selector  Commented=on  InputPortWidth=3  IndexOptions=Index vector (dialog)  Indices=[1]  OutputSizes=1
  Sqrt : Sqrt
  Sum of Elements : Sum  Inputs=+
  Switch : Switch  Threshold=0.5  SaturateOnIntegerOverflow=off  InputSameDT=off
  Terminator : Terminator  Commented=on
  Transpose : Math  Commented=on  Operator=transpose  SignedPower=on
  Trigonometric Function1 : Trigonometry  Operator=atan2
  phi0_rad : Constant  Value=phi0_rad  OutDataTypeStr=single
  phi0_rad1 : Constant  Value=gam0_rad  OutDataTypeStr=single
  psi_zero : Constant  Value=psi  OutDataTypeStr=single
  psi_zero1 : Constant  Commented=on  Value=psi  OutDataTypeStr=single
  quat_0 : Outport  PortDimensions=4
  wires:
  Gain2/1 -> Add2/2
  phi0_rad1/1 -> Add2/1
  phi0_rad/1 -> Add1/1
  Asin/1 -> Add1/2
  Radians to Degrees/1 -> Display/1
  Data Type Conversion/1 -> Scope/1
  Switch/1 -> quat_0/1, Scope1/1
  Magnetic declination1/1 -> Switch/2, Data Type Conversion/1
  Degrees to Radians/1 -> Terminator/1
  Degrees to Radians1/1 -> Mux1/1
  Gain1/1 -> Mux/3, Trigonometric Function1/2
  Transpose/1 -> Product/1
  Mux3/1 -> Rotation Angles to Quaternions1/1
  Add/1 -> Mux3/1, Radians to Degrees/1  "psi_calbymag"
  Magnetic declination/1 -> Degrees to Radians/1
  Atan2/1 -> Add/2
  Selector/1 -> Atan2/1  "magE"
  Selector1/1 -> Atan2/2  "magN"
  Product/1 -> Selector1/1, Selector/1  "magNED"
  Magn_mean_B_guess_LPF/1 -> Product/2
  Quaternions to Direction Cosine Matrix/1 -> Transpose/1
  Add2/1 -> Mux1/3, Mux3/3
  Add1/1 -> Mux1/2, Mux3/2
  psi_zero/1 -> Degrees to Radians1/1
  Mux1/1 -> Rotation Angles to Quaternions/1
  Math Function/1 -> Sum of Elements/1
  Mux/1 -> Math Function/1
  Divide/1 -> Asin/1
  Sum of Elements/1 -> Sqrt/1
  Demux/3 -> Gain1/1
  Demux/2 -> Trigonometric Function1/1, Mux/1
  Demux/1 -> Mux/2, Divide/1
  Trigonometric Function1/1 -> Gain2/1
  Deal with zero/1(Out1) -> Divide/2
  Sqrt/1 -> Deal with zero/1(In1)
  accl_mean_B_m/s_LPF/1 -> Demux/1
  Rotation Angles to Quaternions/1 -> Switch/1, Switch/3

== system VB_RIFKF_UWB_INS25/ISUS_RIEKF M1/INS propogation/Init_PVQ/Subsystem ==
  data : Inport
  Buffer : Buffer  N=50  V=49  OutputFrames=off
  Buffer1 : Buffer  N=50  V=49  OutputFrames=off
  Buffer2 : Buffer  N=50  V=49  ic=-g0  OutputFrames=off
  Demux : Demux  Outputs=3
  Mean4 : dspstat3/Mean  run=off  reset_popup=None  directionMode=Entire input  dimension=3  roiEnable=off  roiType=Rectangles  roiPortion=Entire ROI  roiOutput=Individual statistics for each ROI  roiFlag=off  roundingMode=Floor  overflowMode=off  outputDataTypeStr=Inherit: Same as accumulator  outputMin=[]  outputMax=[]  outputLastDataTypeStr=Inherit: Same as accumulator
  Mean5 : dspstat3/Mean  run=off  reset_popup=None  directionMode=Entire input  dimension=3  roiEnable=off  roiType=Rectangles  roiPortion=Entire ROI  roiOutput=Individual statistics for each ROI  roiFlag=off  roundingMode=Floor  overflowMode=off  outputDataTypeStr=Inherit: Same as accumulator  outputMin=[]  outputMax=[]  outputLastDataTypeStr=Inherit: Same as accumulator
  Mean6 : dspstat3/Mean  run=off  reset_popup=None  directionMode=Entire input  dimension=3  roiEnable=off  roiType=Rectangles  roiPortion=Entire ROI  roiOutput=Individual statistics for each ROI  roiFlag=off  roundingMode=Floor  overflowMode=off  outputDataTypeStr=Inherit: Same as accumulator  outputMin=[]  outputMax=[]  outputLastDataTypeStr=Inherit: Same as accumulator
  Scope : Scope  NumInputPorts=2
  Vector Concatenate : Concatenate  NumInputs=3
  mean_data : Outport
  wires:
  data/1 -> Demux/1, Scope/1
  Vector Concatenate/1 -> mean_data/1, Scope/2
  Mean4/1 -> Vector Concatenate/1
  Demux/3 -> Buffer2/1
  Buffer1/1 -> Mean5/1  "fby_buff"
  Demux/1 -> Buffer/1
  Buffer2/1 -> Mean6/1  "fbz_buff"
  Mean5/1 -> Vector Concatenate/2
  Buffer/1 -> Mean4/1  "fbx_buff"
  Demux/2 -> Buffer1/1
  Mean6/1 -> Vector Concatenate/3

== system VB_RIFKF_UWB_INS25/ISUS_RIEKF M1/INS propogation/Init_PVQ/Subsystem1 ==
  data : Inport
  Buffer : Buffer  N=50  V=49  OutputFrames=off
  Buffer1 : Buffer  N=50  V=49  OutputFrames=off
  Buffer2 : Buffer  N=50  V=49  OutputFrames=off
  Demux : Demux  Outputs=3
  Mean4 : dspstat3/Mean  run=off  reset_popup=None  directionMode=Entire input  dimension=3  roiEnable=off  roiType=Rectangles  roiPortion=Entire ROI  roiOutput=Individual statistics for each ROI  roiFlag=off  roundingMode=Floor  overflowMode=off  outputDataTypeStr=Inherit: Same as accumulator  outputMin=[]  outputMax=[]  outputLastDataTypeStr=Inherit: Same as accumulator
  Mean5 : dspstat3/Mean  run=off  reset_popup=None  directionMode=Entire input  dimension=3  roiEnable=off  roiType=Rectangles  roiPortion=Entire ROI  roiOutput=Individual statistics for each ROI  roiFlag=off  roundingMode=Floor  overflowMode=off  outputDataTypeStr=Inherit: Same as accumulator  outputMin=[]  outputMax=[]  outputLastDataTypeStr=Inherit: Same as accumulator
  Mean6 : dspstat3/Mean  run=off  reset_popup=None  directionMode=Entire input  dimension=3  roiEnable=off  roiType=Rectangles  roiPortion=Entire ROI  roiOutput=Individual statistics for each ROI  roiFlag=off  roundingMode=Floor  overflowMode=off  outputDataTypeStr=Inherit: Same as accumulator  outputMin=[]  outputMax=[]  outputLastDataTypeStr=Inherit: Same as accumulator
  Vector Concatenate : Concatenate  NumInputs=3
  mean_data : Outport
  wires:
  Mean6/1 -> Vector Concatenate/3
  Demux/2 -> Buffer1/1
  Buffer/1 -> Mean4/1  "fbx_buff"
  Mean5/1 -> Vector Concatenate/2
  Buffer2/1 -> Mean6/1  "fbz_buff"
  Demux/1 -> Buffer/1
  Buffer1/1 -> Mean5/1  "fby_buff"
  Demux/3 -> Buffer2/1
  Mean4/1 -> Vector Concatenate/1
  Vector Concatenate/1 -> mean_data/1
  data/1 -> Demux/1

== system VB_RIFKF_UWB_INS25/ISUS_RIEKF M1/INS propogation/Init_PVQ/Subsystem2 ==
  Degrees to Radians1 : simulink_extras/Transformations/Degrees to Radians
  Degrees to Radians2 : simulink_extras/Transformations/Degrees to Radians
  Degrees to Radians3 : simulink_extras/Transformations/Degrees to Radians
  Mux : Mux  Inputs=3
  Rotation Angles to Quaternions : sharedtransform/Rotation Angles to Quaternions  rotationOrder=ZYX  aMode=aMode
  phi : Constant  Value=0.11  OutDataTypeStr=single
  psi_zero : Constant  Value=psi  OutDataTypeStr=single
  theta : Constant  Value=1.17  OutDataTypeStr=single
  Quat0 : Outport
  wires:
  Degrees to Radians1/1 -> Mux/1
  Rotation Angles to Quaternions/1 -> Quat0/1
  phi/1 -> Degrees to Radians2/1
  Mux/1 -> Rotation Angles to Quaternions/1
  theta/1 -> Degrees to Radians3/1
  psi_zero/1 -> Degrees to Radians1/1
  Degrees to Radians3/1 -> Mux/2
  Degrees to Radians2/1 -> Mux/3

== system VB_RIFKF_UWB_INS25/ISUS_RIEKF M1/INS propogation/accl bias compensation/error compensation1 ==
  dda : Inport
  QGC_init : Inport  Port=2
  Add3 : Sum
  Delay : Delay  DelayLength=1  InitialCondition=zeros(3,1)  ExternalReset=Level hold
      settings: InputPortMap=u0,r5
  da : Outport
  wires:
  Add3/1 -> Delay/1, da/1
  QGC_init/1 -> Delay/2
  dda/1 -> Add3/1
  Delay/1 -> Add3/2

== system VB_RIFKF_UWB_INS25/ISUS_RIEKF M1/INS propogation/gyro bias compensation/error compensation ==
  ddg : Inport
  Enable : Inport  Port=2
  QGC_init : Inport  Port=3
  Add3 : Sum
  Delay : Delay  DelayLength=1  InitialCondition=zeros(3,1)  ExternalReset=Level hold
      settings: InputPortMap=u0,r5
  If Action Subsystem1 : Subsystem  TreatAsAtomicUnit=on
  If1 : If  IfExpression=u1 == 1  ShowElse=off
  Scope : Scope
  dg : Outport
  wires:
  QGC_init/1 -> Delay/2
  ddg/1 -> Add3/1
  Add3/1 -> dg/1, Delay/1
  Delay/1 -> Add3/2
  If1/1 -> If Action Subsystem1/Action
  Enable/1 -> If1/1, Scope/1

== system VB_RIFKF_UWB_INS25/ISUS_RIEKF M1/INS propogation/vel//pos update/Kinematic Equation ==
  Cbn : Inport
  Ab : Inport  Port=2
  Add : Sum  Inputs=+-
  Add1 : Sum  Inputs=+-
  Constant : Constant  Value=[0 0 -g0]  OutDataTypeStr=single
  Constant1 : Constant  Value=[0 0 -g0]  OutDataTypeStr=single
  Product : Product  Multiplication=Matrix(*)  RndMeth=Zero
  Product1 : Product  Multiplication=Matrix(*)  RndMeth=Zero
  Scope : Scope
  Scope1 : Scope  NumInputPorts=2
  Transpose : Math  Operator=transpose
  An : Outport
  ab_nog : Outport  Port=2
  wires:
  Add1/1 -> ab_nog/1  "ab_nog"
  Product1/1 -> Add1/2  "gb"
  Constant1/1 -> Product1/2  "gn"
  Transpose/1 -> Product1/1  "Cnb"
  Constant/1 -> Add/2
  Product/1 -> Add/1, Scope/1
  Ab/1 -> Scope1/1, Add1/1, Product/2
  Add/1 -> Scope1/2, An/1
  Cbn/1 -> Product/1, Transpose/1

== system VB_RIFKF_UWB_INS25/ISUS_RIEKF M1/INS propogation/vel//pos update/pos update ==
  dtheta : Inport
  vel_k : Inport  Port=2
  dp : Inport  Port=3
  QGC_init : Inport  Port=4
  p0 : Inport  Port=5
  Add1 : Sum
  Delay1 : Delay  DelayLength=1  InitialConditionSource=Input port  ExternalReset=Rising
      settings: InputPortMap=u0,r5,p4
  Gain1 : Gain  Gain=dt
  MATLAB Function : MATLAB Function  TreatAsAtomicUnit=on
  Reshape1 : Reshape  OutputDimensionality=Column vector (2-D)
  p_k : Outport
  wires:
  MATLAB Function/1(pos_correct) -> p_k/1, Delay1/1
  Add1/1 -> MATLAB Function/3(pos)
  dp/1 -> MATLAB Function/2(KFState_dp)
  dtheta/1 -> MATLAB Function/1(dtheta)
  vel_k/1 -> Gain1/1
  Gain1/1 -> Add1/1
  Delay1/1 -> Add1/2
  Reshape1/1 -> Delay1/3
  QGC_init/1 -> Delay1/2
  p0/1 -> Reshape1/1

== system VB_RIFKF_UWB_INS25/ISUS_RIEKF M1/INS propogation/vel//pos update/vel update ==
  dtheta : Inport
  QGC_init : Inport  Port=2
  An : Inport  Port=3
  KFState_dv : Inport  Port=4
  v0 : Inport  Port=5
  Add : Sum
  Delay : Delay  DelayLength=1  InitialConditionSource=Input port  ExternalReset=Rising
      settings: InputPortMap=u0,r5,p4
  Gain : Gain  Gain=dt
  MATLAB Function : MATLAB Function  TreatAsAtomicUnit=on
  Reshape : Reshape  OutputDimensionality=Column vector (2-D)
  vel_k : Outport
  wires:
  MATLAB Function/1(vel_correct) -> vel_k/1, Delay/1
  Add/1 -> MATLAB Function/3(vel)
  dtheta/1 -> MATLAB Function/1(dtheta)
  KFState_dv/1 -> MATLAB Function/2(KFState_dv)
  Delay/1 -> Add/2
  Gain/1 -> Add/1
  v0/1 -> Reshape/1
  An/1 -> Gain/1
  Reshape/1 -> Delay/3
  QGC_init/1 -> Delay/2
